simulink model "Frequency_logchirp"  (R2021b)
settings: Solver=ode4  StartTime=0.0  StopTime=310  FixedStep=0.02  RelTol=1e-3
settings Model: Creator=Tara.Aryal  LastModifiedBy=Tara.Aryal
settings RTWCC: GenCodeOnly=on  PackageGeneratedCodeAndArtifacts=on  PackageName=logcode.zip
settings CodeAppCC: MaxIdLength=50
settings GRTTargetCC: CombineOutputUpdateFcns=off

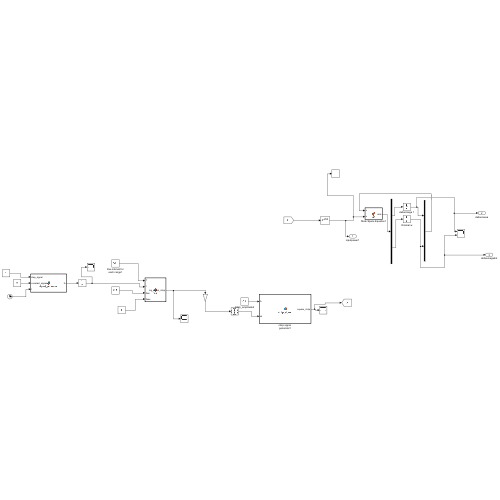
[thumbnail: Simulink's stored preview of the top-level diagram]
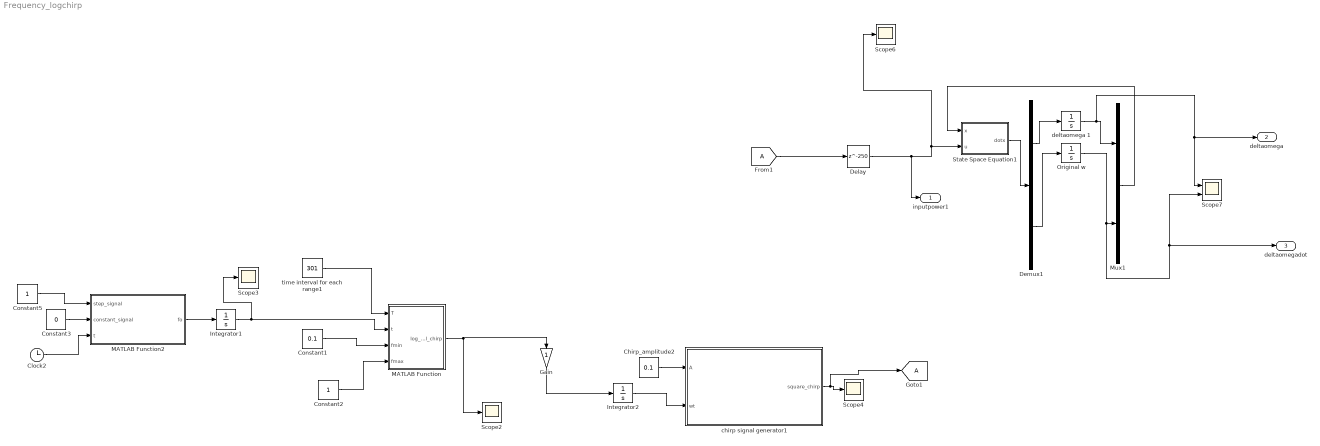
== system Frequency_logchirp ==
  Chirp_amplitude2 : Constant  Value=0.1
  Clock2 : Clock
  Constant1 : Constant  Value=0.1
  Constant2 : Constant
  Constant3 : Constant  Value=0
  Constant5 : Constant
  Delay : Delay  DelayLength=250
  Demux1 : Demux  Outputs=2
  Gain : Gain
  Integrator1 : Integrator
  Integrator2 : Integrator  InitialCondition=0.1  WrapState=on  WrappedStateUpperValue=2*pi  WrappedStateLowerValue=0.0001
  MATLAB Function : MATLAB Function  TreatAsAtomicUnit=on
  MATLAB Function2 : MATLAB Function  TreatAsAtomicUnit=on
  Mux1 : Mux  Inputs=2
  Original w : Integrator
  Scope{2..4,6} (4 alike) : Scope
  Scope7 : Scope  NumInputPorts=2
  State Space Equation1 : MATLAB Function  TreatAsAtomicUnit=on
  chirp signal generator1 : MATLAB Function  TreatAsAtomicUnit=on
  deltaomega 1 : Integrator
  time interval for each range1 : Constant  Value=301
  inputpower1 : Outport
  deltaomega : Outport  Port=2
  deltaomegadot : Outport  Port=3
  tag scope: A=global
  wires:
  time interval for each range1/1 -> MATLAB Function/1(T)
  MATLAB Function/1(log_signal_chirp) -> Gain/1, Scope2/1
  Integrator1/1 -> MATLAB Function/2(t), Scope3/1
  Constant5/1 -> MATLAB Function2/1(step_signal)
  Clock2/1 -> MATLAB Function2/3(t)
  Constant3/1 -> MATLAB Function2/2(constant_signal)
  MATLAB Function2/1(fo) -> Integrator1/1
  Chirp_amplitude2/1 -> chirp signal generator1/1(A)
  Gain/1 -> Integrator2/1
  Integrator2/1 -> chirp signal generator1/2(wt)
  chirp signal generator1/1(square_chirp) -> [A], Scope4/1
  Constant1/1 -> MATLAB Function/3(fmin)
  Constant2/1 -> MATLAB Function/4(fmax)
  Demux1/1 -> deltaomega 1/1
  Delay/1 -> inputpower1/1, Scope6/1, State Space Equation1/2(u)
  Mux1/1 -> State Space Equation1/1(x)
  deltaomega 1/1 -> deltaomega/1, Scope7/1, Mux1/1
  Demux1/2 -> Original w/1
  Original w/1 -> Mux1/2, Scope7/2, deltaomegadot/1
  State Space Equation1/1(dotx) -> Demux1/1
  [A] -> Delay/1

== matlab function Frequency_logchirp/MATLAB Function ==
  data: T input; log_signal_chirp output; t input; fmin input; fmax input
function log_signal_chirp = fcn(T,t, fmin, fmax)
k = floor(t/T);
f0 = fmin;
f1 = fmax;
lambda1 = 1/T * log10(f1 / f0);

log_signal_chirp = f0*(10^(lambda1*(t-k*T)));

== matlab function Frequency_logchirp/State Space Equation1 ==
  data: x input; u input; dotx output
function dotx  = fcn(x, u)
D = 1.5/100;
M = 3.0;
    Tg = 0.2;
    Rp = 0.05;
    Ki=2;
    dotx = zeros(2, 1);
    %x1 = x(1);
    x1 = x(1);
    x2=x(2);
    dotx = [x2;-(D/(M*Tg)+1/(Rp*M*Tg))*x1-(D/M+1/Tg)*x2-1/(M*Tg)*u];

== matlab function Frequency_logchirp/MATLAB Function2 ==
  data: step_signal input; constant_signal input; fo output; t input
function fo   = signal_generator(step_signal,constant_signal,t)

if t <= 0
    fo = constant_signal;
else
    fo = step_signal;
end

== matlab function Frequency_logchirp/chirp signal generator1 ==
  data: square_chirp output; A input; wt input
function square_chirp  = chirp_signal(A,wt)
%quadratic chirp signal


% %square chirp signal generator
% f1=w/(2*pi);
% T = 1/f1;
% k2 = floor(t/T);
% 
% if t > (k2*T) && t< (k2+D)*T
%      square_chirp=1;
% else
%     square_chirp=0;
% end


square_chirp = A*sign(cos(wt));
